simulink subsystem "StudentTemplate_SNGKHA008_M2_sim"  (R2025b)
settings: Solver=VariableStepAuto  StartTime=0.0  StopTime=10.0  RelTol=1e-3
libraries: simulink x3, eeGeneralControl x3
(part 1 of 2)
settings Model: Creator=JesseJabezArendse  LastModifiedBy=muner

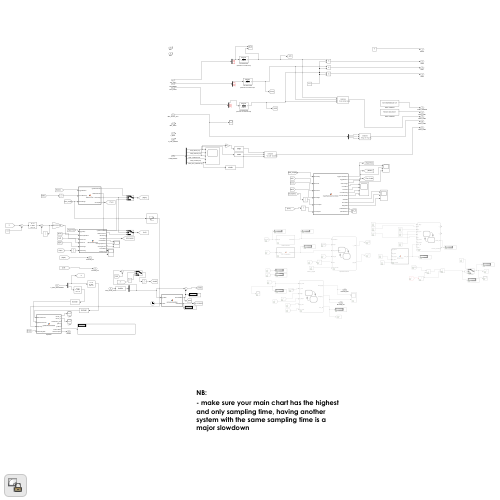
[thumbnail: Simulink's stored preview of the top-level diagram]
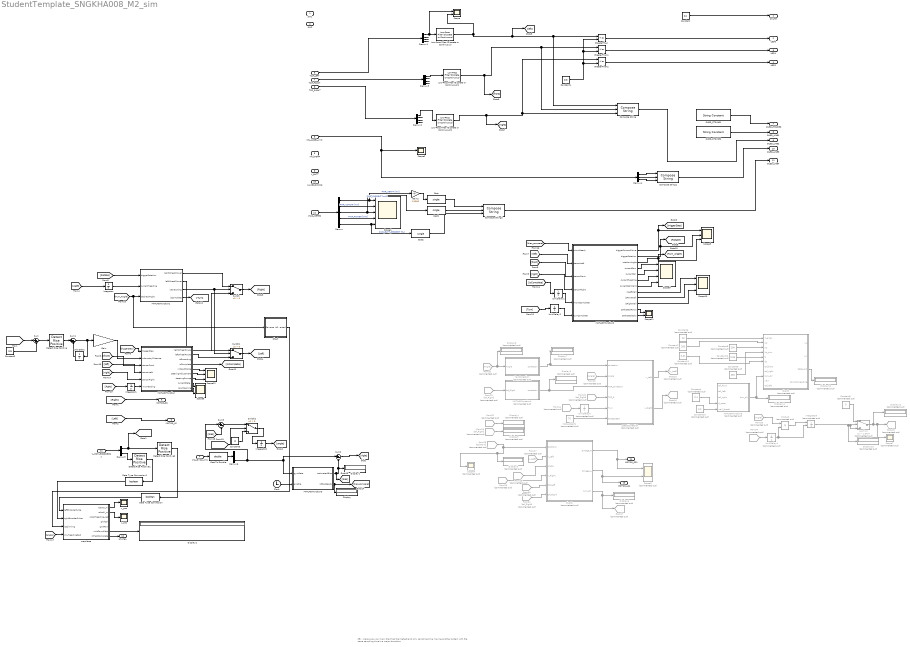
== system StudentTemplate_SNGKHA008_M2_sim ==
  note: NB:
      |
      | - make sure your main chart has the highest and only sampling time, having another system with the same sampling time is a major slowdown
  SW1 : Inport
  SW2 : Inport  Port=2
  IMU_ACCEL_XYZ : Inport  Port=3
  IMU_GYRO_XYZ : Inport  Port=4
  IMU_TEMP : Inport  Port=5
  TOF_LEFT : Inport  Port=6
  TOF_FRONT : Inport  Port=7
  TOF_RIGHT : Inport  Port=8
  V_BATT : Inport  Port=9
  V_LINE_DOWNs : Inport  Port=10
  V_MOT_ENCODERSs : Inport  Port=11
  PWR_METER : Inport  Port=12
  Cast : DataTypeConversion  OutDataTypeStr=single  SaturateOnIntegerOverflow=off  RndMeth=Floor
  Cast To Double : DataTypeConversion  OutDataTypeStr=double  SaturateOnIntegerOverflow=off  RndMeth=Floor
  Cast1 : DataTypeConversion  OutDataTypeStr=single  SaturateOnIntegerOverflow=off  RndMeth=Floor
  Cast2 : DataTypeConversion  OutDataTypeStr=single  SaturateOnIntegerOverflow=off  RndMeth=Floor
  Chart : Stateflow chart  TreatAsAtomicUnit=on
  Chart1 : Stateflow chart  Commented=on  TreatAsAtomicUnit=on
  Chart2 : Stateflow chart  Commented=on  TreatAsAtomicUnit=on
  Clock : Clock
  Compose String : ComposeString  Format="\"L%1.2f F%1.2f R%1.2f\""
  Compose String1 : ComposeString  Format="\"X%2.1f  Y%2.1f  Z%2.1f\""
  Compose String2 : ComposeString  Format="\"%1.2fV  %3.0fmA  %2.0f%%\""
  Constant : Constant  Value=11
  Constant1 : Constant  Value=0.3  SampleTime=-1
  Constant10 : Constant  Commented=on  Value=0.2
  Constant11 : Constant  Commented=on  Value=0.01
  Constant12 : Constant  Commented=on  Value=0.05
  Constant2 : Constant  Value=0.5
  Constant3 : Constant  Value=0
  Constant4 : Constant  Commented=on  Value=0.4
  Constant5 : Constant  Commented=on  Value=0
  Constant6 : Constant  Commented=on  Value=10
  Constant7 : Constant  Commented=on  Value=200
  Constant8 : Constant  Commented=on  Value=200
  Constant9 : Constant  Commented=on  Value=250
  Data Type Conversion : DataTypeConversion  OutDataTypeStr=boolean  SaturateOnIntegerOverflow=off  RndMeth=Floor
  Data Type Conversion1 : DataTypeConversion  OutDataTypeStr=boolean  SaturateOnIntegerOverflow=off  RndMeth=Floor
  Demux : Demux  Outputs=5
  Demux1 : Demux
  Demux2 : Demux
  Demux3 : Demux
  Demux4 : Demux  Outputs=3
  Demux5 : Demux  Outputs=2
  Demux6 : Demux  Outputs=3
  Detect Rise Positive : simulink/Logic and Bit Operations/Detect Rise Positive  vinit=0  OutDataTypeStr=uint8
  Detect Rise Positive1 : simulink/Logic and Bit Operations/Detect Rise Positive  vinit=0  OutDataTypeStr=uint8
  Detect Rise Positive2 : simulink/Logic and Bit Operations/Detect Rise Positive  vinit=0  OutDataTypeStr=uint8
  Display : Display
  Display1 : Display
  Display{3..13} (11 alike) : Display  Commented=on
  Display2 : Display
  From{20,23,26,31} (4 alike) : From  Commented=on  GotoTag=tof_Right
  From21 : From  Commented=on  GotoTag=Angle
  From22 : From  Commented=on  GotoTag=Angle
  From24 : From  Commented=on  GotoTag=turn_dir
  From25 : From  Commented=on  GotoTag=tof_Front
  From27 : From  Commented=on  GotoTag=v_Left
  From28 : From  Commented=on  GotoTag=v_Right
  From29 : From  Commented=on  GotoTag=intAngle
  From30 : From  Commented=on  GotoTag=tof_Left
  From32 : From  Commented=on  GotoTag=tof_Left
  From33 : From  Commented=on  GotoTag=Angle
  From34 : From  Commented=on  GotoTag=turn_dir
  Gain : Gain  Gain=(2*pi*0.031)/8  OutDataTypeStr=double
  Gain2 : Gain  Gain=1/1000
  Goto15 : Goto  Commented=on  GotoTag=v_Left
  Goto16 : Goto  Commented=on  GotoTag=v_Right
  Goto17 : Goto  Commented=on  GotoTag=turn_dir
  Goto18 : Goto  Commented=on  GotoTag=intAngle
  GreaterThan : RelationalOperator  Operator=<=  OutDataTypeStr=boolean  RndMeth=Simplest  InputSameDT=off
  GreaterThan1 : RelationalOperator  Operator=<=  OutDataTypeStr=boolean  RndMeth=Simplest  InputSameDT=off
  GreaterThan2 : RelationalOperator  Operator=<=  OutDataTypeStr=boolean  RndMeth=Simplest  InputSameDT=off
  Integrator : Integrator
  Integrator1 : Integrator
  Integrator2 : Integrator
  Integrator3 : Integrator  Commented=on  ExternalReset=rising  IgnoreLimit=on
  Low-Pass Filter (Discrete or Continuous) : eeGeneralControl/Low-Pass Filter (Discrete or Continuous)  K=1  T=0.1  B=inf  A=-inf  init_option=Inherited from block input  x0=0  Ts=-1
  Low-Pass Filter (Discrete or Continuous)1 : eeGeneralControl/Low-Pass Filter (Discrete or Continuous)  K=1  T=0.1  B=inf  A=-inf  init_option=Inherited from block input  x0=0  Ts=-1
  Low-Pass Filter (Discrete or Continuous)2 : eeGeneralControl/Low-Pass Filter (Discrete or Continuous)  K=1  T=0.1  B=inf  A=-inf  init_option=Inherited from block input  x0=0  Ts=-1
  MATLAB Function : MATLAB Function  TreatAsAtomicUnit=on
  MATLAB Function1 : MATLAB Function  TreatAsAtomicUnit=on
  MATLAB Function2 : MATLAB Function  TreatAsAtomicUnit=on
  MATLAB Function3 : MATLAB Function  TreatAsAtomicUnit=on
  MATLAB Function4 : MATLAB Function  Commented=on  TreatAsAtomicUnit=on
  MATLAB Function5 : MATLAB Function  Commented=on  TreatAsAtomicUnit=on
  Motor_Right1 : Constant  Commented=on  Value=70
  OLED_STRING1 : StringConstant  String="\"UCT MICROMOUSE '25\""
  OLED_STRING2 : StringConstant  String="\"Simulink Data Demo\""
  Product : Product  Commented=on
  Scope : Scope  NumInputPorts=2
      settings: ActiveDisplayYMinimum=0.22759  ActiveDisplayYMaximum=0.52326
  Scope1 : Scope  NumInputPorts=5
      settings: ActiveDisplayYMinimum=-437.5  ActiveDisplayYMaximum=3937.5  DataLoggingVariableName=ScopeData2
  Scope10 : Scope  NumInputPorts=3
      settings: ActiveDisplayYMinimum=0.98925625787217453  ActiveDisplayYMaximum=0.99681786366496772  DataLoggingVariableName=ScopeData10
  Scope11 : Scope  NumInputPorts=2
      settings: ActiveDisplayYMinimum=-0.23906863330343775  ActiveDisplayYMaximum=4.8444494296796581  DataLoggingVariableName=ScopeData11
  Scope12 : Scope  NumInputPorts=3
      settings: ActiveDisplayYMinimum=-2.531731349223886  ActiveDisplayYMaximum=1.0800580317827295  DataLoggingVariableName=ScopeData12
  Scope2 : Scope
  Scope3 : Scope  Commented=on  NumInputPorts=2
      settings: ActiveDisplayYMinimum=3.7629222666728168  ActiveDisplayYMaximum=58.174461604760253  DataLoggingVariableName=ScopeData7  DataLoggingSaveFormat=Array
  Scope4 : Scope  Commented=on
      settings: DataLoggingVariableName=ScopeData8  DataLoggingSaveFormat=Array
  Scope5 : Scope  NumInputPorts=3
      settings: ActiveDisplayYMinimum=0.99964425322969275  ActiveDisplayYMaximum=0.9999942157758529  DataLoggingVariableName=ScopeData5
  Scope6 : Scope  NumInputPorts=2
      settings: ActiveDisplayYMinimum=0.85509125291869592  ActiveDisplayYMaximum=2.7298807987704121  DataLoggingVariableName=ScopeData6
  Scope7 : Scope  Commented=on
      settings: ActiveDisplayYMinimum=-0.42413182902128876  ActiveDisplayYMaximum=1.7667040811774113  DataLoggingVariableName=ScopeData13  DataLoggingSaveFormat=Array
  Scope9 : Scope  NumInputPorts=4
      settings: ActiveDisplayYMinimum=0.35938212114718482  ActiveDisplayYMaximum=4.7848118188048927  DataLoggingVariableName=ScopeData9
  Sum : Sum  Inputs=|+-
  Sum1 : Sum  Inputs=|++
  Sum2 : Sum  Inputs=|+-
  Sum3 : Sum  Inputs=|+-
  Switch : Switch  Criteria=u2 > Threshold  SaturateOnIntegerOverflow=off  InputSameDT=off
  Switch1 : Switch  Criteria=u2 > Threshold  SaturateOnIntegerOverflow=off  InputSameDT=off
  Switch2 : Switch  Criteria=u2 > Threshold  SaturateOnIntegerOverflow=off  InputSameDT=off
  Unit Delay : UnitDelay  SampleTime=-1  HasFrameUpgradeWarning=on
  Unit Delay1 : UnitDelay  SampleTime=-1  HasFrameUpgradeWarning=on
  Unit Delay2 : UnitDelay  SampleTime=-1  HasFrameUpgradeWarning=on
  Unit Delay3 : UnitDelay  Commented=on  SampleTime=-1  HasFrameUpgradeWarning=on
  Unit Delay4 : UnitDelay  Commented=on  SampleTime=-1  HasFrameUpgradeWarning=on
  YawCorrection : Subsystem  Commented=on
  mapMaze : MATLAB Function  TreatAsAtomicUnit=on
  speedCorrection : Stateflow chart  Commented=on  TreatAsAtomicUnit=on
  x_pos : Scope
      settings: ActiveDisplayYMinimum=-0.86826347305388651  ActiveDisplayYMaximum=1.6467065868263511  DataLoggingVariableName=ScopeData4
  y_pos : Scope
      settings: ActiveDisplayYMinimum=0.29695243955776018  ActiveDisplayYMaximum=0.40218354928423572  DataLoggingVariableName=ScopeData3
  yawTurn : Switch  Commented=on  Criteria=u2 > Threshold  Threshold=1.5707  SaturateOnIntegerOverflow=off  InputSameDT=off
  STATE : Outport
  LED0 : Outport  Port=2
  LED1 : Outport  Port=3
  LED2 : Outport  Port=4
  MOTOR_LS : Outport  Port=5
  MOTOR_RS : Outport  Port=6
  OLED_HEADER : Outport  Port=7
  OLED_LINE1 : Outport  Port=8
  OLED_LINE2 : Outport  Port=9
  OLED_LINE3 : Outport  Port=10
  OLED_LINE4 : Outport  Port=11
  STATE1 : Outport  Port=12
  MOTOR_LS1 : Outport  Port=13
  MOTOR_RS1 : Outport  Port=14
  wires:
  TOF_FRONT/1 -> Demux3/1
  OLED_STRING2/1 -> OLED_LINE1/1
  Demux2/1 -> Low-Pass Filter (Discrete or Continuous)2/1
  Demux2/3 -> ?
  Demux2/2 -> ?
  Demux2/4 -> ?
  Compose String1/1 -> OLED_LINE3/1
  GreaterThan1/1 -> LED1/1
  Demux3/3 -> ?
  TOF_RIGHT/1 -> Demux2/1
  Demux3/4 -> ?
  Demux3/2 -> ?
  Demux1/2 -> ?
  Demux3/1 -> Low-Pass Filter (Discrete or Continuous)1/1
  OLED_STRING1/1 -> OLED_HEADER/1
  Demux1/1 -> Scope/1, Low-Pass Filter (Discrete or Continuous)/1
  Compose String/1 -> OLED_LINE2/1
  Constant1/1 -> GreaterThan2/2, GreaterThan1/2, GreaterThan/2
  Demux1/4 -> ?
  GreaterThan2/1 -> LED2/1
  TOF_LEFT/1 -> Demux1/1
  GreaterThan/1 -> LED0/1
  Demux1/3 -> ?
  PWR_METER/1 -> Demux/1
  Demux/1 -> Scope1/1, Gain2/1  "PWR_VBATT [mV]"
  Demux/2 -> Scope1/2  "PWR_VSHUNT [mV]"
  Demux/3 -> Scope1/3, Cast1/1  "PWR_CURRENT [mA]"
  Demux/4 -> Scope1/4  "PWR_POWER [mW]"
  Demux/5 -> Scope1/5, Cast2/1  "PWR_BATT_PERCENT [%]"
  IMU_ACCEL_XYZ/1 -> Demux4/1, Scope2/1
  Demux4/1 -> Compose String1/1
  Demux4/2 -> Compose String1/2
  Demux4/3 -> Compose String1/3
  Compose String2/1 -> OLED_LINE4/1
  Gain2/1 -> Cast/1
  Cast/1 -> Compose String2/1
  Cast1/1 -> Compose String2/2
  Cast2/1 -> Compose String2/3
  Constant/1 -> STATE/1
  Demux5/2 -> Detect Rise Positive1/1
  Demux5/1 -> [Right_encoder], Detect Rise Positive2/1
  V_MOT_ENCODERSs/1 -> Demux5/1
  Sum2/1 -> [Agle]
  MATLAB Function3/2(isBiasReady) -> [bias_compare], Display/1
  MATLAB Function3/1(estimatedBias) -> Sum2/2, Display1/1, [bias]
  Clock/1 -> MATLAB Function3/2(enable)
  [Left] -> MOTOR_LS/1
  [Right] -> MOTOR_RS/1
  [front] -> MATLAB Function/3(sensorFront)
  MATLAB Function1/3(isExecuting) -> Switch/2, Switch1/2
  Integrator1/1 -> MATLAB Function/6(imuHeading)
  [Agle] -> Integrator1/1
  [bias_compare] -> MATLAB Function2/1(isImuReady)
  MATLAB Function/9(sawOpening) -> Scope6/2
  MATLAB Function/6(steeringAdjustment) -> Scope12/2
  Unit Delay1/1 -> MATLAB Function2/5(moveComplete)
  MATLAB Function/5(inCoastMode) -> Scope12/1
  Switch/1 -> [Right]
  MATLAB Function2/12(pathStackCols) -> Scope11/2
  Sum1/1 -> Gain/1, Unit Delay/1
  [isComplete] -> Unit Delay1/1
  [left] -> MATLAB Function/4(sensorLeft)
  [Rotate] -> MATLAB Function1/1(triggerRotation)
  [Turn_Angle] -> MATLAB Function1/3(desiredAngle), Chart/1(Reverse)
  [left] -> MATLAB Function2/2(sensorLeft)
  MATLAB Function/8(currentState) -> Scope6/1
  MATLAB Function2/10(isRightWall) -> Scope10/3
  MATLAB Function/1(rightWheelPower) -> Switch/3
  MATLAB Function2/6(currentHeading) -> Scope9/3
  [Right_encoder] -> Sum/1
  MATLAB Function2/7(currentCellWalls) -> Scope9/4
  [Agle] -> Integrator/1
  Gain/1 -> MATLAB Function/2(odometryDistance)
  [Turn] -> Unit Delay2/1
  MATLAB Function/2(leftWheelPower) -> Switch1/3
  MATLAB Function2/8(isLeftWall) -> Scope10/1
  Constant2/1 -> Sum/2
  MATLAB Function2/5(currentCol) -> Scope9/2
  MATLAB Function/4(isComplete) -> [isComplete]
  MATLAB Function2/3(rotationAngle) -> Scope5/3, [Turn_Angle]
  MATLAB Function2/11(pathStackRows) -> Scope11/1
  Integrator/1 -> MATLAB Function1/2(currentHeading)
  Unit Delay/1 -> Sum1/2
  [front] -> MATLAB Function2/3(sensorFront)
  Sum/1 -> Detect Rise Positive/1
  [right] -> MATLAB Function2/4(sensorRight)
  MATLAB Function1/4(isComplete) -> [Turn]
  Switch1/1 -> [Left]
  MATLAB Function2/9(isFrontWall) -> Scope10/2
  MATLAB Function1/2(leftWheelPower) -> Switch1/1
  MATLAB Function2/2(triggerRotation) -> Scope5/2, [Rotate]
  [right] -> MATLAB Function/5(sensorRight)
  MATLAB Function/7(steeringSource) -> Scope12/3
  MATLAB Function2/1(triggerForwardMove) -> Scope5/1, [triggerStep]
  MATLAB Function1/1(rightWheelPower) -> Switch/1
  [triggerStep] -> MATLAB Function/1(triggerStep)
  Unit Delay2/1 -> MATLAB Function2/6(turnComplete)
  MATLAB Function2/4(currentRow) -> Scope9/1
  Low-Pass Filter (Discrete or Continuous)/1 -> Scope/2, [left], Compose String/1, GreaterThan/1
  Low-Pass Filter (Discrete or Continuous)1/1 -> [front], Compose String/2, GreaterThan1/1
  Low-Pass Filter (Discrete or Continuous)2/1 -> [right], Compose String/3, GreaterThan2/1
  mapMaze/1(robotX_m) -> x_pos/1
  mapMaze/2(robotY_m) -> y_pos/1
  mapMaze/6(visitCountMap) -> Display2/1
  mapMaze/7(isTaskComplete) -> STATE1/1
  Detect Rise Positive/1 -> Sum1/1
  [angle] -> mapMaze/4(imuHeadingRad)
  Integrator2/1 -> [angle]
  Detect Rise Positive2/1 -> Data Type Conversion/1
  Data Type Conversion/1 -> mapMaze/1(leftEncoderPulse)
  Detect Rise Positive1/1 -> Data Type Conversion1/1
  Data Type Conversion1/1 -> mapMaze/2(rightEncoderPulse)
  Chart/1(isReversed) -> mapMaze/3(isSpinning)
  IMU_GYRO_XYZ/1 -> Cast To Double/1
  Cast To Double/1 -> Demux6/1
  Demux6/3 -> Sum2/1, MATLAB Function3/1(gyroRate), Sum3/1
  Sum3/1 -> Switch2/1
  [bias] -> Sum3/2
  Constant3/1 -> Switch2/3
  [bias_compare] -> Switch2/2
  Switch2/1 -> Integrator2/1
  Motor_Right1/1 -> speedCorrection/6(baseSpeed)
  MATLAB Function4/1(correction) -> Display9/1, speedCorrection/3(TOF_correction)
  From23/1 -> MATLAB Function4/1(tof_Right)
  From24/1 -> Unit Delay3/1
  Unit Delay3/1 -> speedCorrection/5(Turn)
  From20/1 -> speedCorrection/4(TOF_R)
  From22/1 -> speedCorrection/2(Angle)
  From21/1 -> Display8/1, YawCorrection/1(Angle)
  YawCorrection/1(correction) -> Display7/1, speedCorrection/1(correction)
  speedCorrection/2(v_Right) -> Goto16/1
  speedCorrection/1(v_Left) -> Goto15/1
  From26/1 -> Display5/1
  From30/1 -> Chart1/5(tof_Left)
  Chart1/2(Omega_L) -> MOTOR_LS1/1, Scope3/2
  Chart1/1(Omega_R) -> Scope3/1, MOTOR_RS1/1
  From28/1 -> Chart1/4(v_Right)
  From25/1 -> Scope4/1, Display3/1, Chart1/1(tof_Front)
  Chart1/3(turn_dir) -> Goto17/1, Display6/1
  From32/1 -> Display4/1
  From27/1 -> Chart1/2(v_Left)
  From31/1 -> Chart1/6(tof_Right)
  From29/1 -> Chart1/3(Angle)
  Constant7/1 -> Chart2/2(Kd)
  Chart2/3(state_out) -> Display10/1
  Constant4/1 -> MATLAB Function5/4(d_open)
  Constant10/1 -> MATLAB Function5/5(wall_thresh)
  MATLAB Function5/1(turn_dir) -> Display11/1, Chart2/9(turn_dir)
  Integrator3/1 -> Display13/1, yawTurn/2, yawTurn/3
  Product/1 -> Integrator3/1
  Constant6/1 -> Chart2/1(K_align)
  Constant8/1 -> Chart2/3(Kp)
  Constant12/1 -> Chart2/5(b)
  From34/1 -> Unit Delay4/1
  From33/1 -> Product/1
  Constant5/1 -> yawTurn/1
  yawTurn/1 -> Display12/1, Scope7/1, Goto18/1
  Unit Delay4/1 -> Product/2, Integrator3/2
  Constant11/1 -> Chart2/6(dt)
  Constant9/1 -> Chart2/4(Kp_turn)

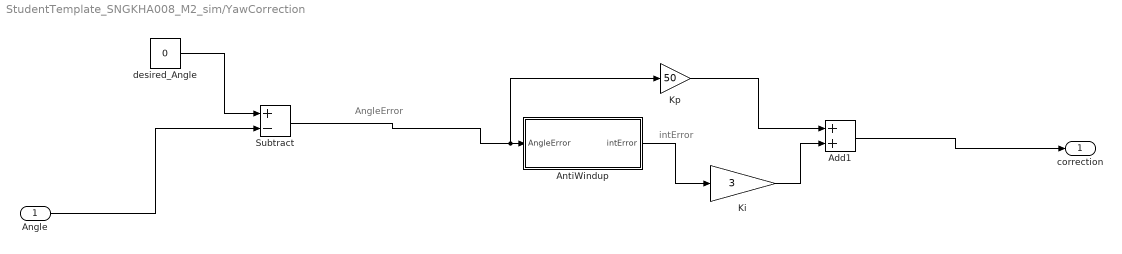
== system StudentTemplate_SNGKHA008_M2_sim/YawCorrection ==
  note: intError
  note: AngleError
  Angle : Inport
  Add1 : Sum
  AntiWindup : MATLAB Function  TreatAsAtomicUnit=on
  Ki : Gain  Gain=3
  Kp : Gain  Gain=50
  Subtract : Sum  Inputs=+-
  desired_Angle : Constant  Value=0
  correction : Outport
  wires:
  desired_Angle/1 -> Subtract/1
  Subtract/1 -> Kp/1, AntiWindup/1(AngleError)
  Add1/1 -> correction/1
  Angle/1 -> Subtract/2
  Kp/1 -> Add1/1
  AntiWindup/1(intError) -> Ki/1
  Ki/1 -> Add1/2

== matlab function StudentTemplate_SNGKHA008_M2_sim/MATLAB Function1 ==
  settings: updateMethod=DISCRETE
  data: triggerRotation input; rightWheelPower output; currentHeading input; desiredAngle input; leftWheelPower output; isExecuting output; isComplete output
function [rightWheelPower, leftWheelPower, isExecuting, isComplete] = executeTurn( ...
    triggerRotation, currentHeading, desiredAngle)
%#codegen
% Rotate a specified angle (radians) using integrated heading input.
% Adds: decel profile near target, overshoot micro-brake, settle window.
% ---------- Tunables ----------
MAX_ROTATION_SPEED         = 55;                 % full spin power far from target
MIN_ROTATION_SPEED         = 18;                 % stiction floor near target
DECELERATION_THRESHOLD_RAD = deg2rad(35);        % begin ramping down inside this
SETTLE_TOLERANCE_IN_RAD  = deg2rad(1.0);       % must get inside this to start settle
HYSTERESIS_TOLERANCE_RAD = deg2rad(1.5);       % hysteresis: if error grows past this, keep turning
SETTLE_DURATION_TICKS    = uint8(6);           % how long to hold inside band
OVERSHOOT_BRAKE_POWER    = 22;                 % brief opposite-sign tap after overshoot
BRAKE_DURATION_TICKS     = uint8(4);           % duration of the tap
% ---------- Cast ----------
currentHeading = double(currentHeading);
desiredAngle = double(desiredAngle);
triggerEdge  = (triggerRotation ~= 0);
% ---------- Persistent state ----------
persistent currentState isRotating initialHeading isReady settleTimer brakeTimer previousErrorSign
% currentState: 0=idle, 1=spinning, 2=braking, 3=settling
if isempty(isRotating)
    isRotating        = false;
    initialHeading    = 0.0;
    isReady           = true;
    currentState      = uint8(0);
    settleTimer       = uint8(0);
    brakeTimer        = uint8(0);
    previousErrorSign = 0;
end
% ---------- Defaults ----------
rightWheelPower = 0.0;
leftWheelPower  = 0.0;
isExecuting     = 0.0;
isComplete      = 0.0;
% ---------- Start edge ----------
if ~isRotating && isReady && triggerEdge
    isRotating        = true;
    initialHeading    = currentHeading;
    isReady           = false;
    currentState      = uint8(1);   % start in spinning
    settleTimer       = uint8(0);
    brakeTimer        = uint8(0);
    previousErrorSign = 0;
end
% Rearm when idle and command low
if (~triggerEdge) && ~isReady && ~isRotating
    isReady = true;
end
% ---------- Helper: compute power with decel profile ----------
    function [powerLevel, direction, errorRad, absErrorRad] = calculate_rotation_power()
        % remaining angle (positive => need CCW)
        errorRad    = desiredAngle - (currentHeading - initialHeading);
        absErrorRad = abs(errorRad);
        direction    = sign(errorRad); if direction==0, direction=1; end
        if absErrorRad >= DECELERATION_THRESHOLD_RAD
            powerLevel = MAX_ROTATION_SPEED;
        else
            % Linear ramp from DECELERATION_THRESHOLD_RAD down to stiction floor
            rampFactor = absErrorRad / max(DECELERATION_THRESHOLD_RAD, 1e-9);
            powerLevel   = MIN_ROTATION_SPEED + (MAX_ROTATION_SPEED - MIN_ROTATION_SPEED)*rampFactor;
        end
    end
% ---------- State machine ----------
if isRotating
    switch currentState
        case 1 % actively spinning
            [powerLevel, direction, errorRad, absErrorRad] = calculate_rotation_power();
            % Detect crossing past target (sign flip)
            currentErrorSign = sign(errorRad); if currentErrorSign==0, currentErrorSign = previousErrorSign; end
            overshotTarget = (previousErrorSign ~= 0) && (currentErrorSign ~= 0) && (currentErrorSign ~= previousErrorSign);
            previousErrorSign = currentErrorSign;
            % If inside the enter band, move to settle
            if absErrorRad <= SETTLE_TOLERANCE_IN_RAD
                currentState    = uint8(3); % settling
                settleTimer     = SETTLE_DURATION_TICKS;
                leftWheelPower  = 0.0; rightWheelPower = 0.0;
                isExecuting     = 1.0;
                % no return; let the bottom return once per tick
            % If we crossed, do a brief brake
            elseif overshotTarget
                currentState    = uint8(2);   % braking
                brakeTimer      = BRAKE_DURATION_TICKS;
                % brake is opposite sign of previous command, i.e., -direction
                leftWheelPower  =  -OVERSHOOT_BRAKE_POWER * (-direction);
                rightWheelPower =   OVERSHOOT_BRAKE_POWER * (-direction);
                isExecuting     = 1.0;
                return;
            else
                % Normal spin with decel + stiction floor
                leftWheelPower  =  -max(MIN_ROTATION_SPEED, powerLevel) * direction;
                rightWheelPower =   max(MIN_ROTATION_SPEED, powerLevel) * direction;
                isExecuting     = 1.0;
                return;
            end
        case 2 % braking (short reverse tap to kill momentum)
            if brakeTimer > 0
                % Keep applying opposite sign to current error
                % Recompute direction from fresh error:
                errorRad = desiredAngle - (currentHeading - initialHeading);
                direction = sign(errorRad); if direction==0, direction=1; end
                leftWheelPower  =  -OVERSHOOT_BRAKE_POWER * (-direction);
                rightWheelPower =   OVERSHOOT_BRAKE_POWER * (-direction);
                isExecuting     = 1.0;
                brakeTimer      = brakeTimer - 1;
                return;
            else
                % After brake, go back to spinning to finish precisely
                currentState = uint8(1);
            end
        case 3 % settling inside tolerance band
            errorRad    = desiredAngle - (currentHeading - initialHeading);
            absErrorRad = abs(errorRad);
            if absErrorRad <= HYSTERESIS_TOLERANCE_RAD
                % hold zero power and count down
                leftWheelPower  = 0.0; rightWheelPower = 0.0;
                isExecuting     = 1.0;
                if settleTimer > 0
                    settleTimer = settleTimer - 1;
                end
                if settleTimer == 0
                    % success
                    isComplete  = 1.0;
                    isExecuting = 0.0;
                    isRotating  = false;
                    currentState  = uint8(0);
                end
                return;
            else
                % drifted back out of band → resume spinning
                currentState = uint8(1);
                % fall-through to compute a new spin command this tick:
                [powerLevel, direction] = calculate_rotation_power();
                leftWheelPower  =  -max(MIN_ROTATION_SPEED, powerLevel) * direction;
                rightWheelPower =   max(MIN_ROTATION_SPEED, powerLevel) * direction;
                isExecuting     = 1.0;
                return;
            end
    end
end
% If we get here and not spinning, stay idle
% (defaults already zero)
end

== matlab function StudentTemplate_SNGKHA008_M2_sim/MATLAB Function ==
  settings: updateMethod=DISCRETE
  data: triggerStep input; rightWheelPower output; odometryDistance input; sensorFront input; sensorLeft input; sensorRight input; imuHeading input; leftWheelPower output; isExecuting output; isComplete output; inCoastMode output; steeringAdjustment output; steeringSource output; currentState output; sawOpening output
function [rightWheelPower, leftWheelPower, isExecuting, isComplete, inCoastMode, steeringAdjustment, steeringSource, currentState, sawOpening] = advanceOneCell( ...
    triggerStep, odometryDistance, sensorFront, sensorLeft, sensorRight, imuHeading)
%#codegen
% Move forward one "cell" with wall-centering using TOF.
% Priority: Safety stop → Coast-to-wall → Opening-glide → Normal motion → Hold.
% Opening-glide uses the same steering correction helper (not forced gyro).
% ===== Tunables =====
CELL_DISTANCE      = 0.194;     % [m]
BASE_SPEED         = 85;        % base forward command
FRONT_STOP_THRESHOLD = 0.055;     % [m] hard stop threshold
% Side-wall centering
P_GAIN_BOTH_WALLS  = 1200.0;
P_GAIN_ONE_WALL    = 1200.0;
SETPOINT_LEFT_WALL   = 0.076;     % [m]
SETPOINT_RIGHT_WALL  = 0.076;     % [m]
MAX_STEERING_ADJUST  = 120.0;
SIDE_SENSOR_MIN_RANGE = 0.00;
SIDE_SENSOR_MAX_RANGE = 0.10;
% Gyro heading-hold (used only when no walls in calculate_steering)
P_GAIN_YAW           = 800.0;    % motor delta per rad yaw error
MAX_YAW_ADJUST       = 120.0;
% Post-distance hold
POST_MOVE_DURATION   = uint16(55); % ticks
POST_MOVE_SPEED      = 35;
%% --- COAST TO WALL (front TOF) ---
ALLOW_FRONT_COAST    = true;
COAST_TRIGGER_FRACTION = 0.7;
COAST_TRIGGER_DISTANCE = 0.15;       % [m] if sensorFront < this and > FRONT_STOP_THRESHOLD → coast
COAST_SPEED          = 65;
%% --- OPENING DETECTION (side TOF jump up) ---
OPENING_DELTA_METERS   = 0.05;         % [m] increase over gap means "opening"
OPENING_DETECT_LOOKBACK = uint8(3);     % compare current to N ticks ago
SENSOR_HISTORY_SIZE     = uint8(16);    % history buffer length (> OPENING_DETECT_LOOKBACK)
OPENING_GLIDE_DURATION = uint16(215);  % ticks to roll into opening before stopping
OPENING_GLIDE_SPEED    = 65;
% ===== Cast numerics =====
odometryDistance = double(odometryDistance);
sensorFront  = double(sensorFront);
sensorLeft   = double(sensorLeft);
sensorRight  = double(sensorRight);
imuHeading   = double(imuHeading);
% ===== Persistent state =====
persistent isDriving initialOdometry isReady isHoldingPosition holdTimer ...
           initialHeading isCoastingToWall isGlidingPastOpening ...
           openingGlideTimer leftHistory rightHistory historyIndex
if isempty(isDriving)
    isDriving             = false;
    initialOdometry       = 0.0;
    isReady               = true;
    isHoldingPosition     = false;
    holdTimer             = uint16(0);
    initialHeading        = 0.0;
    isCoastingToWall      = false;
    isGlidingPastOpening  = false;
    openingGlideTimer     = uint16(0);
    leftHistory = SETPOINT_LEFT_WALL  * ones(1, double(SENSOR_HISTORY_SIZE));
    rightHistory = SETPOINT_RIGHT_WALL * ones(1, double(SENSOR_HISTORY_SIZE));
    historyIndex = uint8(1);
end
% ===== Defaults =====
rightWheelPower = 0; leftWheelPower = 0;
isExecuting = 0.0; isComplete = 0.0; inCoastMode = 0.0;
steeringAdjustment = 0.0; steeringSource = 0.0;
currentState = 0.0; sawOpening = 0.0;
% ===== History update (with NaN hold) =====
nextHistoryIndex = uint8( 1 + mod(double(historyIndex), double(SENSOR_HISTORY_SIZE)) );
currentHistoryIndex = historyIndex;
currentLeft = sensorLeft;  if isnan(currentLeft),  currentLeft  = leftHistory(double(currentHistoryIndex)); end
currentRight = sensorRight; if isnan(currentRight),  currentRight  = rightHistory(double(currentHistoryIndex)); end
leftHistory(double(nextHistoryIndex)) = currentLeft;
rightHistory(double(nextHistoryIndex)) = currentRight;
historyIndex = nextHistoryIndex;
    function historyValue = get_history_value(historyBuffer, ticksAgo)
        lookbackIndex = 1 + mod(double(historyIndex)-1 - double(ticksAgo), double(SENSOR_HISTORY_SIZE));
        historyValue = historyBuffer(lookbackIndex);
    end
% ===== Start a new move =====
if ~isDriving && ~isHoldingPosition && ~isCoastingToWall && ~isGlidingPastOpening && isReady && (triggerStep ~= 0)
    isDriving         = true;
    initialOdometry   = odometryDistance;
    initialHeading    = imuHeading;
    isReady           = false;
end
% ===== Re-arm when fully idle =====
if (triggerStep == 0) && ~isReady && ~isDriving && ~isHoldingPosition && ~isCoastingToWall && ~isGlidingPastOpening
    isReady = true;
end
% ===== Safety stop =====
if (~isnan(sensorFront)) && (sensorFront <= FRONT_STOP_THRESHOLD)
    rightWheelPower = 0; leftWheelPower = 0;
    isExecuting = 0.0; isComplete = 1.0; inCoastMode = double(isCoastingToWall);
    steeringAdjustment = 0.0; steeringSource = 0.0; currentState = 0.0; sawOpening = 0.0;
    isDriving = false; isHoldingPosition = false; isCoastingToWall = false; isGlidingPastOpening = false;
    holdTimer = uint16(0); openingGlideTimer = uint16(0);
    return;
end
% ===== Steering correction helper =====
    function [adjustment, source] = calculate_steering()
        isLeftSensorValid  = (~isnan(sensorLeft))  && (sensorLeft  >= SIDE_SENSOR_MIN_RANGE) && (sensorLeft  <= SIDE_SENSOR_MAX_RANGE);
        isRightSensorValid = (~isnan(sensorRight)) && (sensorRight >= SIDE_SENSOR_MIN_RANGE) && (sensorRight  <= SIDE_SENSOR_MAX_RANGE);
        if isLeftSensorValid && isRightSensorValid
            wallDifferenceSetpoint = SETPOINT_LEFT_WALL - SETPOINT_RIGHT_WALL;
            adjustment = P_GAIN_BOTH_WALLS * ((sensorLeft - sensorRight) - wallDifferenceSetpoint);
            source = 2;
        elseif isLeftSensorValid
            adjustment = P_GAIN_ONE_WALL * (sensorLeft - SETPOINT_LEFT_WALL);
            source = 1;
        elseif isRightSensorValid
            adjustment = -P_GAIN_ONE_WALL * (sensorRight - SETPOINT_RIGHT_WALL);
            source = 1;
        else
            headingError = mod((imuHeading - initialHeading) + pi, 2*pi) - pi;
            adjustment   = -P_GAIN_YAW * headingError;
            if adjustment >  MAX_YAW_ADJUST, adjustment =  MAX_YAW_ADJUST; end
            if adjustment < -MAX_YAW_ADJUST, adjustment = -MAX_YAW_ADJUST; end
            source = 3;
        end
        if adjustment >  MAX_STEERING_ADJUST, adjustment =  MAX_STEERING_ADJUST; end
        if adjustment < -MAX_STEERING_ADJUST, adjustment = -MAX_STEERING_ADJUST; end
    end
%% ===== PHASE 1: COAST TO WALL =====
if isCoastingToWall
    currentState = 1.0; inCoastMode = 1.0; sawOpening = double(isGlidingPastOpening);
    basePower = COAST_SPEED;
    [steerAdjust, steerSource] = calculate_steering();
    steeringAdjustment = steerAdjust; steeringSource = double(steerSource);
    rightWheelPower = basePower + steerAdjust;
    leftWheelPower  = basePower - steerAdjust;
    isExecuting = 1.0;
    return;
end
%% ===== PHASE 2: OPENING GLIDE (pre-emptable by Phase 1) =====
if isGlidingPastOpening
    % Allow Phase 1 to override immediately
    if ~isnan(sensorFront) && (sensorFront < COAST_TRIGGER_DISTANCE) && (sensorFront > FRONT_STOP_THRESHOLD)
        isGlidingPastOpening = false;
        isCoastingToWall     = true;
        isDriving            = false;
        isHoldingPosition    = false;
        currentState   = 1.0; inCoastMode = 1.0; sawOpening = 0.0;
        basePower      = COAST_SPEED;
        [steerAdjust, steerSource] = calculate_steering();
        steeringAdjustment = steerAdjust; steeringSource = double(steerSource);
        rightWheelPower = basePower + steerAdjust; leftWheelPower  = basePower - steerAdjust;
        isExecuting     = 1.0;
        return;
    end
    % Continue opening glide
    currentState = 2.0; sawOpening = 1.0;
    basePower = OPENING_GLIDE_SPEED;
    [steerAdjust, steerSource] = calculate_steering();
    steeringAdjustment = steerAdjust; steeringSource = double(steerSource);
    rightWheelPower = basePower + steerAdjust; leftWheelPower  = basePower - steerAdjust;
    isExecuting = 1.0;
    if openingGlideTimer > 0
        openingGlideTimer = openingGlideTimer - 1;
    end
    if openingGlideTimer == 0
        % === EXIT BLOCK IMMEDIATELY WHEN GLIDE FINISHES ===
        isGlidingPastOpening = false; sawOpening = 0.0;
        isDriving = false; isHoldingPosition = false; isCoastingToWall = false;
        rightWheelPower = 0; leftWheelPower = 0;
        isExecuting = 0.0; isComplete = 1.0; currentState = 0.0;
    end
    return;
end
%% ===== PHASE 3: MOVING =====
if isDriving
    currentState = 3.0; sawOpening = 0.0;
    distanceTraveled = odometryDistance - initialOdometry;
    % Opening detection using gap over N ticks ago
    previousLeft = get_history_value(leftHistory, OPENING_DETECT_LOOKBACK);
    previousRight = get_history_value(rightHistory, OPENING_DETECT_LOOKBACK);
    deltaLeft = currentLeft - previousLeft; deltaRight = currentRight - previousRight;
    isOpeningFound = ((deltaLeft >= OPENING_DELTA_METERS) || (deltaRight >= OPENING_DELTA_METERS));
    if distanceTraveled < CELL_DISTANCE
        basePower = BASE_SPEED;
        [steerAdjust, steerSource] = calculate_steering();
        steeringAdjustment = steerAdjust; steeringSource = double(steerSource);
        rightWheelPower = basePower + steerAdjust; leftWheelPower  = basePower - steerAdjust;
        isExecuting = 1.0;
        % Arm coast-to-wall late in the block
        if ALLOW_FRONT_COAST && (distanceTraveled >= COAST_TRIGGER_FRACTION*CELL_DISTANCE)
            if ~isnan(sensorFront) && (sensorFront < COAST_TRIGGER_DISTANCE) && (sensorFront > FRONT_STOP_THRESHOLD)
                isCoastingToWall = true;
            end
        end
        % Start opening-glide if detected and not coasting
        if isOpeningFound && ~isCoastingToWall
            isGlidingPastOpening = true;
            openingGlideTimer    = OPENING_GLIDE_DURATION;
            sawOpening           = 1.0;
            % Prevent later fall-through to HOLD for this block:
            isDriving           = false;
            isHoldingPosition   = false;
        end
    else
        % Past nominal distance: either enter coast-to-wall or hold
        if ALLOW_FRONT_COAST && ~isCoastingToWall && ~isGlidingPastOpening
            if ~isnan(sensorFront) && (sensorFront < COAST_TRIGGER_DISTANCE) && (sensorFront > FRONT_STOP_THRESHOLD)
                isCoastingToWall = true;   % Phase 1 will win next tick
            else
                isDriving         = false;
                isHoldingPosition = true;
                holdTimer         = POST_MOVE_DURATION;
                currentState      = 4.0;
            end
        elseif ~ALLOW_FRONT_COAST && ~isGlidingPastOpening
            isDriving         = false;
            isHoldingPosition = true;
            holdTimer         = POST_MOVE_DURATION;
            currentState      = 4.0;
        end
    end
end
%% ===== PHASE 4: HOLD =====
if isHoldingPosition
    currentState = 4.0; sawOpening = 0.0;
    basePower = POST_MOVE_SPEED;
    [steerAdjust, steerSource] = calculate_steering();
    steeringAdjustment = steerAdjust; steeringSource = double(steerSource);
    rightWheelPower = basePower + steerAdjust; leftWheelPower  = basePower - steerAdjust;
    isExecuting = 1.0;
    if holdTimer > 0
        holdTimer = holdTimer - 1;
    end
    if holdTimer == 0
        rightWheelPower = 0; leftWheelPower = 0;
        isExecuting = 0.0; isComplete = 1.0;
        isHoldingPosition = false;
        currentState = 0.0;
    end
end
end
